simulink model "USV_2DOF_SS_tcurve_SURGE_wPID_FF"  (R2015b)
settings: Solver=VariableStepAuto  StartTime=0.0  StopTime=45  RelTol=1e-3
values from neighbouring files (symbols this model uses):
  breakpoints1 = data(end:-1:1,1)'    [FEB02_LAKE_TEST.m]    (also in GainIteration_Coup.m; load_tcurve_table.m)
  Kd = Gain(3,i)    [YawModelGains.m]
  Kp = Gain(1,i)    [YawModelGains.m]
  switch_1 = switch_case(i)    [SurgeModelGains.m]
  table_data = data(end:-1:1,2)'    [FEB02_LAKE_TEST.m]    (also in GainIteration_Coup.m; load_tcurve_table.m)
undefined symbols (not defined in the file or in its folder): Ki
settings Model: Creator=bsb  LastModifiedBy=aschnieders22
settings ConfigComp: CovModelRefEnable=Off
settings ConfigurationSet: Description=Simscape Multibody

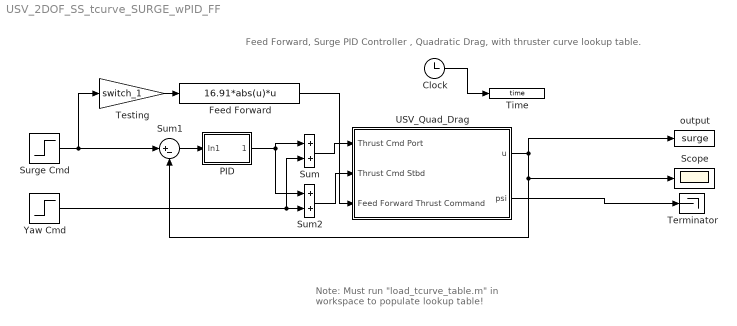
== system USV_2DOF_SS_tcurve_SURGE_wPID_FF ==
  note: Note: Must run "load_tcurve_table.m" in workspace to populate lookup table!
  note: Feed Forward, Surge PID Controller , Quadratic Drag, with thruster curve lookup table.
  Clock : Clock
  Feed Forward : Fcn  Expr=16.91*abs(u)*u
  PID : Subsystem
  Scope : Scope
  Sum : Sum
  Sum1 : Sum  Inputs=|+-
  Sum2 : Sum
  Surge Cmd : Step  Time=10  Before=1.25  After=1.5  SampleTime=0
  Terminator : Terminator
  Testing : Gain  Gain=switch_1
  Time : ToWorkspace  VariableName=time  SampleTime=-1
  USV_Quad_Drag : Subsystem
  Yaw Cmd : Step  After=0  SampleTime=0
  output : ToWorkspace  VariableName=surge  SampleTime=-1
  wires:
  Sum/1 -> USV_Quad_Drag/1(Thrust Cmd Port)
  Sum2/1 -> USV_Quad_Drag/2(Thrust Cmd Stbd)
  USV_Quad_Drag/2(psi) -> Terminator/1
  Sum1/1 -> PID/1(In1)
  Surge Cmd/1 -> Testing/1, Sum1/1
  USV_Quad_Drag/1(u) -> output/1, Sum1/2, Scope/1
  Yaw Cmd/1 -> Sum/2, Sum2/2
  PID/1(Out1) -> Sum2/1, Sum/1
  Feed Forward/1 -> USV_Quad_Drag/3("Feed Forward Thrust Command ")
  Testing/1 -> Feed Forward/1
  Clock/1 -> Time/1

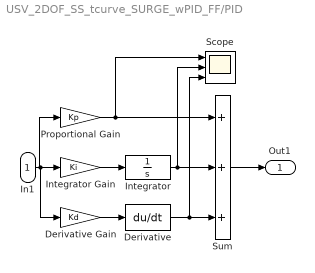
== system USV_2DOF_SS_tcurve_SURGE_wPID_FF/PID ==
  In1 : Inport
  Derivative : Derivative  CoefficientInTFapproximation=0
  Derivative Gain : Gain  Gain=Kd
  Integrator : TransferFcn  Denominator=[1 0]
  Integrator Gain : Gain  Gain=Ki
  Proportional Gain : Gain  Gain=Kp
  Scope : Scope  NumInputPorts=3
  Sum : Sum  Inputs=+++
  Out1 : Outport
  wires:
  Derivative Gain/1 -> Derivative/1
  Integrator Gain/1 -> Integrator/1
  Derivative/1 -> Scope/3, Sum/3
  Sum/1 -> Out1/1
  Integrator/1 -> Scope/2, Sum/2
  Proportional Gain/1 -> Scope/1, Sum/1
  In1/1 -> Derivative Gain/1, Integrator Gain/1, Proportional Gain/1

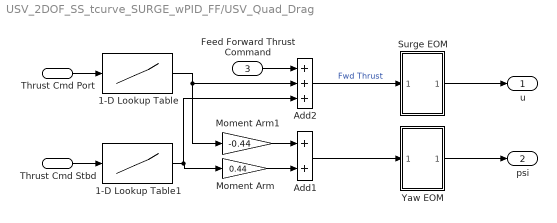
== system USV_2DOF_SS_tcurve_SURGE_wPID_FF/USV_Quad_Drag ==
  Thrust Cmd Port : Inport
  Thrust Cmd Stbd : Inport  Port=2
  "Feed Forward Thrust Command " : Inport  Port=3
  1-D Lookup Table : Lookup_n-D  NumberOfTableDimensions=1  BreakpointsForDimension1=breakpoints1  Table=table_data  ExtrapMethod=Clip  UseLastTableValue=on  InternalRulePriority=Speed  RndMeth=Simplest  InputSameDT=on
  1-D Lookup Table1 : Lookup_n-D  NumberOfTableDimensions=1  BreakpointsForDimension1=breakpoints1  Table=table_data  ExtrapMethod=Clip  UseLastTableValue=on  InternalRulePriority=Speed  RndMeth=Simplest  InputSameDT=on
  Add1 : Sum
  Add2 : Sum  Inputs=+++
  Moment Arm : Gain  Gain=0.44
  Moment Arm1 : Gain  Gain=-0.44
  Surge EOM : Subsystem
  Yaw EOM : Subsystem
  u : Outport
  psi : Outport  Port=2
  wires:
  1-D Lookup Table/1 -> Add2/2, Moment Arm1/1
  Thrust Cmd Port/1 -> 1-D Lookup Table/1
  1-D Lookup Table1/1 -> Add2/3, Moment Arm/1
  Thrust Cmd Stbd/1 -> 1-D Lookup Table1/1
  Moment Arm1/1 -> Add1/1
  Moment Arm/1 -> Add1/2
  Add1/1 -> Yaw EOM/1(In1)
  Yaw EOM/1(Out1) -> psi/1
  Add2/1 -> Surge EOM/1(In1)  "Fwd Thrust"
  Surge EOM/1(Out1) -> u/1
  "Feed Forward Thrust Command "/1 -> Add2/1

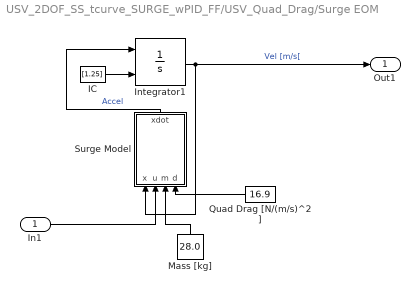
== system USV_2DOF_SS_tcurve_SURGE_wPID_FF/USV_Quad_Drag/Surge EOM ==
  In1 : Inport
  IC : Constant  Value=[1.25]
  Integrator1 : Integrator  InitialConditionSource=external
  Mass [kg] : Constant  Value=28.0
  Quad Drag [N/(m/s)^2] : Constant  Value=16.9
  Surge Model : MATLAB Function  TreatAsAtomicUnit=on
  Out1 : Outport
  wires:
  Integrator1/1 -> Out1/1, Surge Model/1(x)  "Vel [m/s["
  Surge Model/1(xdot) -> Integrator1/1  "Accel"
  In1/1 -> Surge Model/2(u)
  Mass [kg]/1 -> Surge Model/3(m)
  Quad Drag [N/(m/s)^2]/1 -> Surge Model/4(d)
  IC/1 -> Integrator1/2

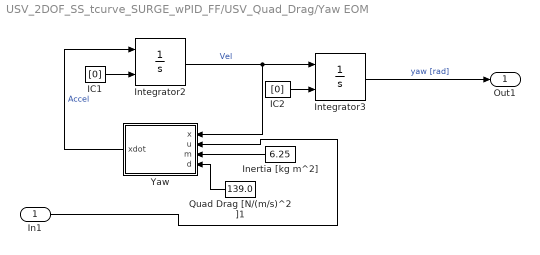
== system USV_2DOF_SS_tcurve_SURGE_wPID_FF/USV_Quad_Drag/Yaw EOM ==
  In1 : Inport
  IC1 : Constant  Value=[0]
  IC2 : Constant  Value=[0]
  Inertia [kg m^2] : Constant  Value=6.25
  Integrator2 : Integrator  InitialConditionSource=external
  Integrator3 : Integrator  InitialConditionSource=external
  Quad Drag [N/(m/s)^2]1 : Constant  Value=139.0
  Yaw : MATLAB Function  TreatAsAtomicUnit=on
  Out1 : Outport
  wires:
  IC1/1 -> Integrator2/2
  IC2/1 -> Integrator3/2
  In1/1 -> Yaw/2(u)
  Yaw/1(xdot) -> Integrator2/1  "Accel"
  Integrator2/1 -> Integrator3/1, Yaw/1(x)  "Vel"
  Inertia [kg m^2]/1 -> Yaw/3(m)
  Quad Drag [N/(m/s)^2]1/1 -> Yaw/4(d)
  Integrator3/1 -> Out1/1  "yaw [rad]"

== matlab function USV_2DOF_SS_tcurve_SURGE_wPID_FF/USV_Quad_Drag/Yaw EOM/Yaw ==
  data: x input; u input; xdot output; m input; d input
function xdot = fcn(x,u,m,d)
%#codegen

% x - state of the system.  surge velocity.
% u - input. thrust force
% Model parameters
m = m; %28.0;   % Mass [kg]
d = d; %16.9;  % Quadratic drag coefficient [N/(m/s)^2]

xdot = 1/m*(-d*abs(x)*x+u);

== matlab function USV_2DOF_SS_tcurve_SURGE_wPID_FF/USV_Quad_Drag/Surge EOM/Surge Model ==
  data: x input; u input; xdot output; m input; d input
function xdot = fcn(x,u,m,d)
%#codegen

% x - state of the system.  surge velocity.
% u - input. thrust force
% Model parameters
m = m; %28.0;   % Mass [kg]
d = d; %16.9;  % Quadratic drag coefficient [N/(m/s)^2]

xdot = 1/m*(-d*abs(x)*x+u);
